simulink model "LinearControlSim"  (R2018b)
settings: Solver=ode1  StartTime=0.0  StopTime=5  FixedStep=0.002  RelTol=1e-3
undefined symbols (not defined in the file or in its folder): A, Am, B, Bm, C, Cm, D, Dm
settings Model: Creator=alexj  LastModifiedBy=alexj

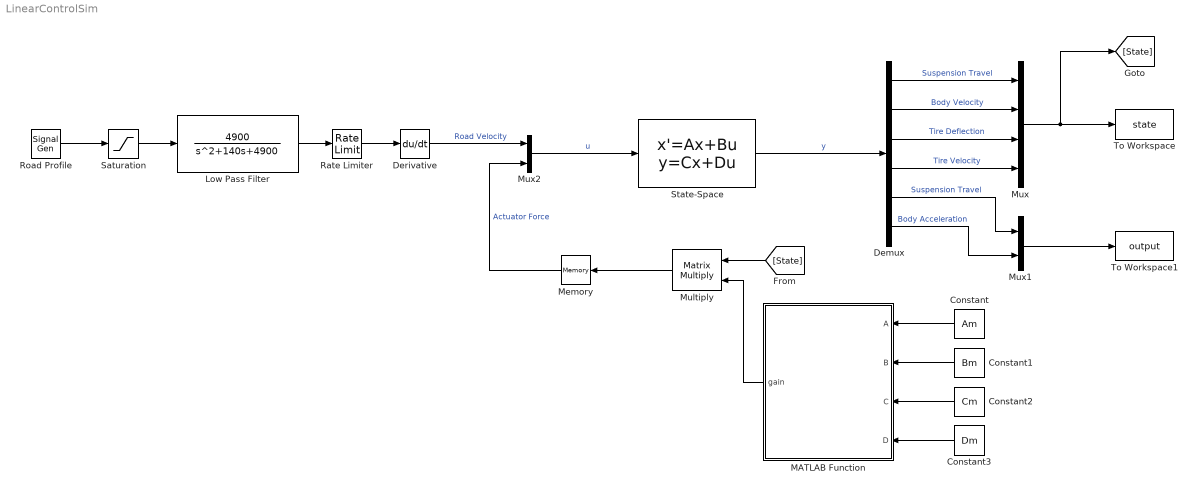
== system LinearControlSim ==
  Constant : Constant  Value=Am
  Constant1 : Constant  Value=Bm
  Constant2 : Constant  Value=Cm
  Constant3 : Constant  Value=Dm
  Demux : Demux  Outputs=6
  Derivative : Derivative
  "Low Pass Filter " : TransferFcn  Numerator=[4900]  Denominator=[1 140 4900]
  MATLAB Function : MATLAB Function  TreatAsAtomicUnit=on
  Memory : Memory
  Multiply : Product  Multiplication=Matrix(*)
  Mux : Mux
  Mux1 : Mux  Inputs=2
  Mux2 : Mux  Inputs=2
  Rate Limiter : RateLimiter  RisingSlewLimit=0.2  FallingSlewLimit=-0.2  SampleTimeMode=inherited
  "Road Profile " : SignalGenerator  WaveForm=square  Amplitude=0.01  Frequency=0.3
  Saturation : Saturate  UpperLimit=1  LowerLimit=-1
  State-Space : StateSpace  A=A  B=B  C=[eye(4);C]  D=[zeros(4,2);D]  InitialCondition=0
  To Workspace : ToWorkspace  VariableName=state  SaveFormat=Timeseries  SampleTime=-1
  To Workspace1 : ToWorkspace  VariableName=output  SaveFormat=Timeseries  SampleTime=-1
  wires:
  Mux2/1 -> State-Space/1  "u"
  State-Space/1 -> Demux/1  "y"
  MATLAB Function/1(gain) -> Multiply/2
  Constant/1 -> MATLAB Function/1(A)
  Constant2/1 -> MATLAB Function/3(C)
  Constant3/1 -> MATLAB Function/4(D)
  Constant1/1 -> MATLAB Function/2(B)
  Demux/1 -> Mux/1  "Suspension Travel"
  Demux/2 -> Mux/2  "Body Velocity"
  Demux/3 -> Mux/3  "Tire Deflection"
  Demux/4 -> Mux/4  "Tire Velocity"
  Demux/6 -> Mux1/2  "Body Acceleration"
  Demux/5 -> Mux1/1  "Suspension Travel"
  Mux/1 -> [State], To Workspace/1
  Mux1/1 -> To Workspace1/1
  "Road Profile "/1 -> Saturation/1
  Saturation/1 -> "Low Pass Filter "/1
  "Low Pass Filter "/1 -> Rate Limiter/1
  Multiply/1 -> Memory/1
  Memory/1 -> Mux2/2  "Actuator Force"
  Rate Limiter/1 -> Derivative/1
  Derivative/1 -> Mux2/1  "Road Velocity"
  [State] -> Multiply/1

== matlab function LinearControlSim/MATLAB Function ==
  data: A input; gain output; B input; C input; D input
function gain = feedbackGain(A, B, C, D)

gain = 0*[1 1 1 1]';
